simulink model "Robot_Control"  (R2016b)
settings: Solver=ode1  StartTime=0.0  StopTime=Inf  FixedStep=0.001  RelTol=1e-3
PostLoadFcn:
  | , if any(exist('dsrtsu_mdlpostloadfcn', 'file') == [2, 3, 6]), try dsrtsu_mdlpostloadfcn('Execute', bdroot); catch fprintf('Error in PostLoadFcn (dsrtsu_mdlpostloadfcn) for model "%s":\n %s\n', bdroot, lasterr); end, end,
libraries: rtiethernetlib x4
settings Model: DSRTSU_INTERNAL_RTI_VER=490  DSRTSU_INTERNAL_RTI_TYPE=rti1202  Creator=labuser  LastModifiedBy=labuser
settings OptimizationCC: BlockReduction=off  ConditionallyExecuteInputs=off  OptimizeBlockIOStorage=off  BufferReuse=off  GlobalBufferReuse=off  ExpressionFolding=off  LocalBlockOutputs=off
settings HardwareCC: ProdBitPerPointer=32  ProdBitPerSizeT=32  ProdBitPerPtrDiffT=32  ProdLargestAtomicInteger=Integer  ProdEndianess=BigEndian  ProdWordSize=32  ProdHWDeviceType=Custom Processor->Custom  TargetIntDivRoundTo=Zero  TargetEndianess=BigEndian  TargetHWDeviceType=Custom Processor->Custom
settings RTWCC: SystemTargetFile=rti1202.tlc  MakeCommand=make_rti  TemplateMakefile=rti1202.tmf  Description=dSPACE DS1202 Hardware Platform
settings STFCustomTargetCC: ParMdlRefBuildCompliant=on  GRTInterface=off  SystemTargetFile=rti1202.tlc
settings GRTTargetCC: TargetLangStandard=C89/C90 (ANSI)  CompOptLevelCompliant=off  ConcurrentExecutionCompliant=off  CombineOutputUpdateFcns=off  MatFileLogging=off  CPPClassGenCompliant=off  UseToolchainInfoCompliant=off
settings ConfigComp: CovMetricSettings=dswe

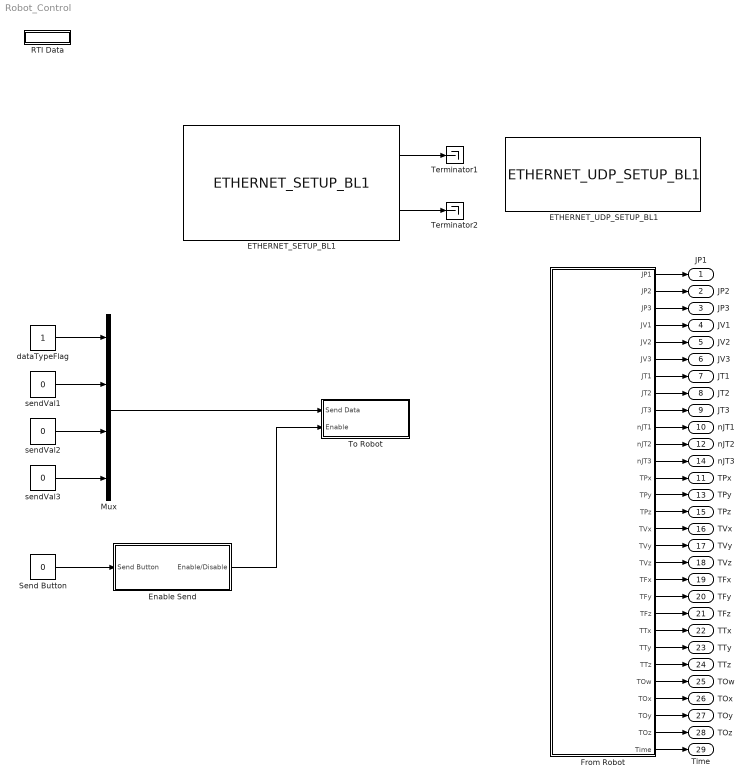
== system Robot_Control ==
  ETHERNET_SETUP_BL1 : rtiethernetlib/ETHERNET_SETUP_BL1  DSProperties=struct('RTI',struct('Version',uint32(2),'BlockType',struct('isSLSource',uint8(0),'isSLSink',uint8(0),'isHWSource',uint8(0),'isHWSink',uint8(0),'isSetup',uint8(1),'isInline',uint8(1),'isNonInline',uint8(0),'isInterrupt',uint8(0),'isChannelwise',uint8(0)),'IOBoardType','DSETHERNET','UnitType','ETHERNET','Identifier','SETUP','DialogType','ML','BlockSet','RTIETHERNET','SlaveProcessor','NONE'))  RTIBlockInterface=struct('OutputPortsWidth',int32([2 1 1 4]),'OutputPortsActive',[0 0 1 1],'OutputPortsName',{{['Link Status'],['Watchdog Status'],['DHCP Status'],['Local IP']}},'OutputPortsDataType',{{'SS_UINT32','SS_UINT32','SS_UINT32','SS_UINT8'}},'InitLevel',3,'IconTransparency','on','BlockDisplay',{{['Ethernet Setup\n\nLocal IP: By DHCP Server'],'left'}},'DialogFcn','rtiethernetsetupgui','BlockName',struct('Token',{{'ETHERNET_SETUP_BL1'}}))  RTIBlockParameters=struct('DHCPserverMode',{{1,'OFF',[0 1]}},'LocalIpNum1',{{'137','OFF',[0 255]}},'LocalIpNum2',{{'148','OFF',[0 255]}},'LocalIpNum3',{{'205','OFF',[0 255]}},'LocalIpNum4',{{'167','OFF',[0 255]}},'SubnetMaskNum1',{{'255','OFF',[0 255]}},'SubnetMaskNum2',{{'255','OFF',[0 255]}},'SubnetMaskNum3',{{'254','OFF',[0 255]}},'SubnetMaskNum4',{{'0','OFF',[0 255]}},'GatewayNum1',{{'0','OFF',[0 255]}},'GatewayNum2',{{'0','OFF',[0 255]}},'GatewayNum3',{{'0','OFF',[0 255]}},'GatewayNum4',{{'0','OFF',[0 255]}},'LinkStatusOutPortMode',{{0,'OFF',[0 1]}},'NumOfEthConnectors',{{2,'ON',[1 16]}},'WatchdogStatusOutPortMode',{{0,'OFF',[0 1]}},'LocalIpOutPortMode',{{1,'OFF',[0 1]}},'IpAndSubmaskCheck',{{int32(0),'OFF',[0 1]}},'TLCFileName',{{'rtiethernetsetup','OFF',[]}})  RTISFcnParameters=struct('DHCPserverMode','int32','LocalIpNum1','uint8','LocalIpNum2','uint8','LocalIpNum3','uint8','LocalIpNum4','uint8','SubnetMaskNum1','uint8','SubnetMaskNum2','uint8','SubnetMaskNum3','uint8','SubnetMaskNum4','uint8','GatewayNum1','uint8','GatewayNum2','uint8','GatewayNum3','uint8','GatewayNum4','uint8','LinkStatusOutPortMode','int32','NumOfEthConnectors','int32','WatchdogStatusOutPortMode','int32','LocalIpOutPortMode','int32','TLCFileName','char')  RTIBlockParaDefault=struct('DHCPserverMode',0,'LocalIpNum1',192,'LocalIpNum2',168,'LocalIpNum3',140,'LocalIpNum4',6,'SubnetMaskNum1',255,'SubnetMaskNum2',255,'SubnetMaskNum3',255,'SubnetMaskNum4',0,'GatewayNum1',0,'GatewayNum2',0,'GatewayNum3',0,'GatewayNum4',0,'LinkStatusOutPortMode',1,'NumOfEthConnectors',3,'WatchdogStatusOutPortMode',0,'LocalIpOutPortMode',0,'IpAndSubmaskCheck',1,'TLCFileName','rtiethernetsetup')
  ETHERNET_UDP_SETUP_BL1 : rtiethernetlib/ETHERNET_UDP_SETUP_BL1  DSProperties=struct('RTI',struct('Version',uint32(2),'BlockType',struct('isSLSource',uint8(1),'isSLSink',uint8(1),'isHWSource',uint8(0),'isHWSink',uint8(0),'isSetup',uint8(0),'isInline',uint8(1),'isNonInline',uint8(0),'isInterrupt',uint8(0),'isChannelwise',uint8(0)),'IOBoardType','DSETHERNET','UnitType','UDP','Identifier','SETUPUDP','DialogType','ML','BlockSet','RTIETHERNET','SlaveProcessor','NONE'))  RTIBlockInterface=struct('OutputPortsWidth',int32(2),'OutputPortsActive',0,'OutputPortsName',{{['RX Dropped Frames']}},'OutputPortsDataType',{{'SS_DOUBLE'}},'InputPortsWidth',int32([4 1]),'InputPortsActive',int32([0 0]),'InputPortsName',{{['RX Remote IP Filter'],['RX Remote Port Filter']}},'InputPortsDataType',{{'SS_UINT8','SS_UINT16'}},'RWork',{{{'RX_DROPPED_FRAMES',uint32(2)}}},'InitLevel',3,'IconTransparency','on','BlockDisplay',{{['Ethernet UDP/IP\nSetup\n\nSocket ID: 0'],'center'}},'DialogFcn','rtiethernetsetupudpgui','BlockName',struct('Token',{{'ETHERNET_UDP_SETUP_BL1'}}))  RTIBlockParameters=struct('SocketId',{{0,'OFF',[]}},'EnableSocketBind',{{1,'OFF',[0 1]}},'AcceptAnyRxRemoteIp',{{1,'OFF',[0 1]}},'RxRemoteIpNum1',{{'172','OFF',[0 255]}},'RxRemoteIpNum2',{{'20','OFF',[0 255]}},'RxRemoteIpNum3',{{'41','OFF',[0 255]}},'RxRemoteIpNum4',{{'226','OFF',[0 255]}},'EnableDynamicRxRemoteIpFilter',{{0,'OFF',[0 1]}},'AcceptAnyRxRemotePort',{{1,'OFF',[0 1]}},'RxRemotePort',{{'9930','OFF',[1 65535]}},'EnableDynamicRxRemotePortFilter',{{0,'OFF',[0 1]}},'TxRemoteIpNum1',{{'137','OFF',[0 255]}},'TxRemoteIpNum2',{{'148','OFF',[0 255]}},'TxRemoteIpNum3',{{'204','OFF',[0 255]}},'TxRemoteIpNum4',{{'55','OFF',[0 255]}},'TxRemotePort',{{'9930','OFF',[1 65535]}},'SpecifyLocalPort',{{1,'OFF',[0 1]}},'LocalPort',{{'9931','OFF',[1 65535]}},'InterruptMode',{{0,'OFF',[0 1]}},'RxDroppedFramesOutPortMode',{{0,'OFF',[0 1]}},'RemoteIpNumCheck',{{0,'OFF',[0 1]}},'RemotePortCheck',{{0,'OFF',[0 1]}},'LocalPortCheck',{{1,'OFF',[0 1]}},'DHCPserverModeEnabled',{{0,'OFF',[0 1]}},'TLCFileName',{{'rtiethernetsetupudp','OFF',[]}})  RTISFcnParameters=struct('SocketId','double','EnableSocketBind','int32','AcceptAnyRxRemoteIp','int32','RxRemoteIpNum1','uint8','RxRemoteIpNum2','uint8','RxRemoteIpNum3','uint8','RxRemoteIpNum4','uint8','EnableDynamicRxRemoteIpFilter','int32','AcceptAnyRxRemotePort','int32','RxRemotePort','uint16','EnableDynamicRxRemotePortFilter','int32','TxRemoteIpNum1','uint8','TxRemoteIpNum2','uint8','TxRemoteIpNum3','uint8','TxRemoteIpNum4','uint8','TxRemotePort','uint16','SpecifyLocalPort','int32','LocalPort','uint16','InterruptMode','int32','RxDroppedFramesOutPortMode','int32','DHCPserverModeEnabled','int32','TLCFileName','char')  RTIBlockParaDefault=struct('SocketId',-1,'EnableSocketBind',1,'AcceptAnyRxRemoteIp',1,'RxRemoteIpNum1',0,'RxRemoteIpNum2',0,'RxRemoteIpNum3',0,'RxRemoteIpNum4',0,'EnableDynamicRxRemoteIpFilter',0,'AcceptAnyRxRemotePort',1,'RxRemotePort',49002,'EnableDynamicRxRemotePortFilter',0,'TxRemoteIpNum1',0,'TxRemoteIpNum2',0,'TxRemoteIpNum3',0,'TxRemoteIpNum4',0,'TxRemotePort',49002,'SpecifyLocalPort',0,'LocalPort',49001,'InterruptMode',0,'RxDroppedFramesOutPortMode',0,'RemoteIpNumCheck',0,'RemotePortCheck',0,'LocalPortCheck',0,'DHCPserverModeEnabled',0,'TLCFileName','rtiethernetsetupudp')
  Enable Send : Subsystem
  From Robot : Subsystem
  Mux : Mux
  RTI Data : Subsystem  Tag=struct('RTIDataServer',struct('RTIDataServerVs','2','RTIModelDescription','struct(''main'',''Robot_Control'',''sub'','''',''isMp'',0)'))  LoadFcn="if exist('rtidc'), try,  rtidc('DataHostBlockClbLoad', gcbh); catch, disp(['Warning: ''LoadFcn'' for RTI Data block failed: ' lasterr]); end, end,"  mask(RTI_DATA_HOST){}
      mask help:
      | RTI Data Block.
      | This block is used by RTI to store internal model-dependent data.
      | Please keep this block on the root level of the model. Deleting this block will result in data loss.
      |
      | NEVER DELETE OR COPY THIS BLOCK!
      settings: CopyFcn="if exist('rtidc'), try,  rtidc('DataHostBlockClbCopy', gcbh); catch, disp(['Warning: ''CopyFcn'' for RTI Data block failed: ' lasterr]); end, end,"  DeleteFcn="if exist('rtidc'), try,  rtidc('DataHostBlockClbDelete', gcbh); catch, disp(['Warning: ''DeleteFcn'' for RTI Data block failed: ' lasterr]); end, end,"  ModelCloseFcn="if exist('rtidc'), try,  rtidc('DataHostBlockClbModelClose', gcbh); catch, disp(['Warning: ''ModelCloseFcn'' for RTI Data block failed: ' lasterr]); end, end,"  PreSaveFcn="if exist('rtidc'), try,  rtidc('DataHostBlockClbPreSave', gcbh); catch, disp(['Warning: ''PreSaveFcn'' for RTI Data block failed: ' lasterr]); end, end,"  PostSaveFcn="if exist('rtidc'), try,  rtidc('DataHostBlockClbPostSave', gcbh); catch, disp(['Warning: ''PostSaveFcn'' for RTI Data block failed: ' lasterr]); end, end,"  NameChangeFcn="if exist('rtidc'), try,  rtidc('DataHostBlockClbNameChange', gcbh); catch, disp(['Warning: ''NameChangeFcn'' for RTI Data block failed: ' lasterr]); end, end,"
      mask Help:
      | RTI Data Block.
      | This block is used by RTI to store internal model-dependent data.
      | Please keep this block on the root level of the model. Deleting this block will result in data loss.
      | 
      | NEVER DELETE OR COPY THIS BLOCK!
      mask Display:
      | text(0.5, 0.5, 'RTI Data', 'HorizontalAlignment', 'center');
      | plot([1 0]);
  Send Button : Constant  Value=0
  Terminator1 : Terminator
  Terminator2 : Terminator
  To Robot : Subsystem
  dataTypeFlag : Constant  Description=|
      | This block determines the data type that the robot controller receives. 
      | If the controller expects a data type different than what you send, it will beep and throw an error.
      | Data Types:
      | 1 - Joint Position
      | 2 - Joint Velocity
      | 3 - Joint Torque (gravity compensated)
      | 4 - Joint Torque (not gravity compensated)
      | 5 - Tool Position
      | 6 - Tool Velocity
  sendVal1 : Constant  Value=0
  sendVal2 : Constant  Value=0
  sendVal3 : Constant  Value=0
  JP1 : Outport
  JP2 : Outport  Port=2
  JP3 : Outport  Port=3
  JV1 : Outport  Port=4
  JV2 : Outport  Port=5
  JV3 : Outport  Port=6
  JT1 : Outport  Port=7
  JT2 : Outport  Port=8
  JT3 : Outport  Port=9
  nJT1 : Outport  Port=10
  TPx : Outport  Port=11
  nJT2 : Outport  Port=12
  TPy : Outport  Port=13
  nJT3 : Outport  Port=14
  TPz : Outport  Port=15
  TVx : Outport  Port=16
  TVy : Outport  Port=17
  TVz : Outport  Port=18
  TFx : Outport  Port=19
  TFy : Outport  Port=20
  TFz : Outport  Port=21
  TTx : Outport  Port=22
  TTy : Outport  Port=23
  TTz : Outport  Port=24
  TOw : Outport  Port=25
  TOx : Outport  Port=26
  TOy : Outport  Port=27
  TOz : Outport  Port=28
  Time : Outport  Port=29
  wires:
  ETHERNET_SETUP_BL1/1 -> Terminator1/1
  ETHERNET_SETUP_BL1/2 -> Terminator2/1
  From Robot/13(TPx) -> TPx/1
  From Robot/14(TPy) -> TPy/1
  From Robot/15(TPz) -> TPz/1
  From Robot/1(JP1) -> JP1/1
  From Robot/2(JP2) -> JP2/1
  From Robot/3(JP3) -> JP3/1
  From Robot/29(Time) -> Time/1
  From Robot/28(TOz) -> TOz/1
  From Robot/27(TOy) -> TOy/1
  From Robot/26(TOx) -> TOx/1
  From Robot/25(TOw) -> TOw/1
  From Robot/24(TTz) -> TTz/1
  From Robot/23(TTy) -> TTy/1
  From Robot/22(TTx) -> TTx/1
  From Robot/21(TFz) -> TFz/1
  From Robot/20(TFy) -> TFy/1
  From Robot/19(TFx) -> TFx/1
  From Robot/18(TVz) -> TVz/1
  From Robot/17(TVy) -> TVy/1
  From Robot/16(TVx) -> TVx/1
  From Robot/12(nJT3) -> nJT3/1
  From Robot/11(nJT2) -> nJT2/1
  From Robot/10(nJT1) -> nJT1/1
  From Robot/9(JT3) -> JT3/1
  From Robot/8(JT2) -> JT2/1
  From Robot/7(JT1) -> JT1/1
  From Robot/6(JV3) -> JV3/1
  From Robot/5(JV2) -> JV2/1
  From Robot/4(JV1) -> JV1/1
  Enable Send/1(Enable/Disable) -> To Robot/2(Enable)
  Send Button/1 -> Enable Send/1(Send Button)
  dataTypeFlag/1 -> Mux/1
  sendVal1/1 -> Mux/2
  sendVal2/1 -> Mux/3
  sendVal3/1 -> Mux/4
  Mux/1 -> To Robot/1(Send Data)

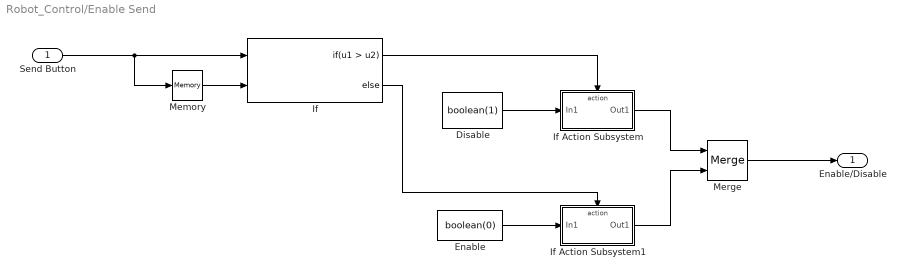
== system Robot_Control/Enable Send ==
  Send Button : Inport
  Disable : Constant  Value=boolean(1)
  Enable : Constant  Value=boolean(0)
  If : If  NumInputs=2  IfExpression=u1 > u2
  If Action Subsystem : Subsystem  TreatAsAtomicUnit=on
  If Action Subsystem1 : Subsystem  TreatAsAtomicUnit=on
  Memory : Memory
  Merge : Merge
  Enable/Disable : Outport
  wires:
  If Action Subsystem1/1(Out1) -> Merge/2
  If/1 -> If Action Subsystem/Action
  If/2 -> If Action Subsystem1/Action
  Send Button/1 -> Memory/1, If/1
  Enable/1 -> If Action Subsystem1/1(In1)
  Memory/1 -> If/2
  Merge/1 -> Enable/Disable/1
  Disable/1 -> If Action Subsystem/1(In1)
  If Action Subsystem/1(Out1) -> Merge/1

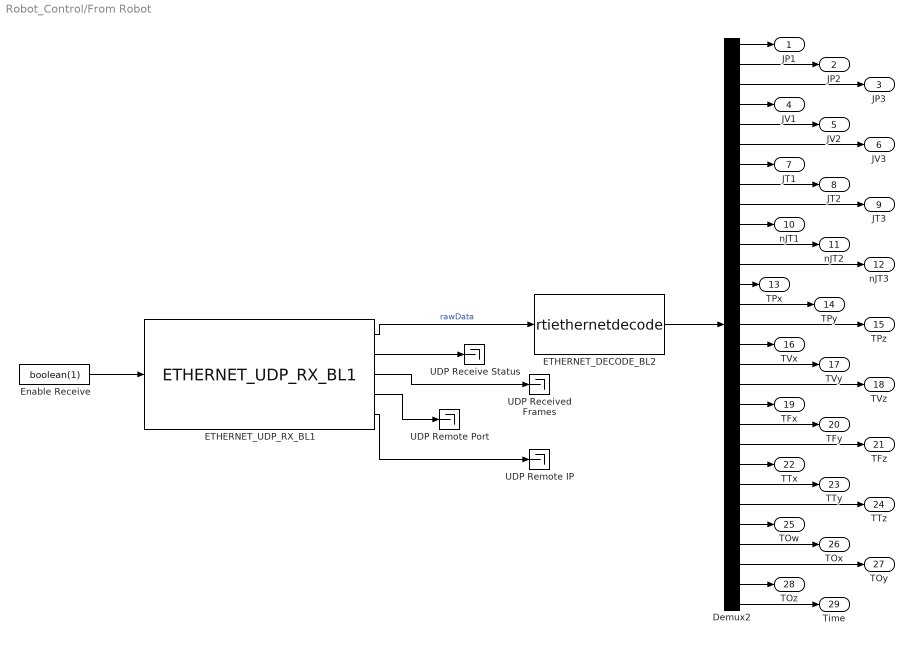
== system Robot_Control/From Robot ==
  Demux2 : Demux  Outputs=29
  ETHERNET_DECODE_BL2 : S-Function  FunctionName=rtiethernetdecode  Parameters=byteordering,offset,auto_offset,datatype,one_datatype,sampletime  SFunctionDeploymentMode=off  EnableBusSupport=off  mask(Ethernet Decode){byteordering=Little endian (Intel), offset=[0], auto_offset=on, datatype=[9 9 9 9 9 9 9 9 9 9 9 9 9 9 9 9 9 9 9 9 9 9 9 9 9 9 9 9 3], one_datatype=off, sampletime=.002}
      mask prompts: byteordering "Byte ordering:"; offset "Offset (bytes):"; auto_offset "Auto offset"; one_datatype "One datatype only"
      mask help:
      | Converts a byte input data stream into the specified datatypes on the output port.
      |
      | Datatype codes:
      | BOOLEAN:  1   //   INT8:      2   //   UINT8:    3
      | INT16  :     4   //   UINT16:  5   //   INT32:     6
      | UINT32 :    7   //   FLOAT:    8   //   DOUBLE:  9
      mask Help: To get further information on this block, refer to the RTI Ethernet blockset documentation.
      mask TypeOptions byteordering: Big endian (Motorola) | Little endian (Intel)
      mask Callback auto_offset: rtiethernetfcnlib('EnableEnDecodeGuiControl', gcbh, 'auto_offset', 2)
      mask Display: text(0.5,0.5, 'Ethernet\nDecode', 'HorizontalAlignment', 'center')
  ETHERNET_UDP_RX_BL1 : rtiethernetlib/ETHERNET_UDP_RX_BL1  DSProperties=struct('RTI',struct('Version',uint32(1),'BlockType',struct('isSLSource',uint8(1),'isSLSink',uint8(1),'isHWSource',uint8(0),'isHWSink',uint8(1),'isSetup',uint8(0),'isInline',uint8(1),'isNonInline',uint8(0),'isInterrupt',uint8(0),'isChannelwise',uint8(0)),'IOBoardType','DSETHERNET','UnitType','UDP','Identifier','RXUDP','DialogType','ML','BlockSet','RTIETHERNET','SlaveProcessor','NONE'))  RTIBlockInterface=struct('OutputPortsWidth',int32([232 1 1 1 4 1]),'OutputPortsActive',[1 1 1 0 1 1],'OutputPortsName',{{'Data','Status',['Received Frames'],['Received Bytes'],['Remote IP'],['Remote Port']}},'OutputPortsDataType',{{'SS_UINT8','SS_UINT32','SS_DOUBLE','SS_UINT32','SS_UINT8','SS_UINT16'}},'InputPortsWidth',int32(1),'InputPortsActive',1,'InputPortsName',{{'Enable'}},'InputPortsDataType',{{'SS_BOOLEAN'}},'RWork',{{{'RECEIVED_FRAMES',uint32(1)}}},'InitLevel',3,'IconTransparency','on','BlockDisplay',{{['Ethernet UDP/IP\nRX\n\nSocket ID: 0'],'center'}},'DialogFcn','rtiethernetrxudpgui','BlockName',struct('Token',{{'ETHERNET_UDP_RX_BL1'}}))  RTIBlockParameters=struct('SocketIdIndex',{{2,'OFF',[1 2]}},'SocketId',{{0,'OFF',[-1 inf]}},'RemoteIp',{{['<NOT AVAILABLE>'],'OFF',[]}},'RemotePort',{{['<NOT AVAILABLE>'],'OFF',[]}},'LocalPort',{{9931,'OFF',[]}},'FrameSize',{{'232','OFF',[1 65507]}},'EnableVariableFrameSize',{{0,'OFF',[0 1]}},'VariableFrameSizeMode',{{1,'OFF',[1 2]}},'InterruptMode',{{0,'OFF',[0 1]}},'RemoteIpOutPortMode',{{1,'OFF',[0 1]}},'RemotePortOutPortMode',{{1,'OFF',[0 1]}},'TLCFileName',{{'rtiethernetrxudp','OFF',[]}})  RTISFcnParameters=struct('SocketIdIndex','int32','SocketId','double','FrameSize','uint16','EnableVariableFrameSize','int32','VariableFrameSizeMode','int32','InterruptMode','int32','RemoteIpOutPortMode','int32','RemotePortOutPortMode','int32','TLCFileName','char')  RTIBlockParaDefault=struct('SocketIdIndex',1,'SocketId',-1,'RemoteIp',['<NOT AVAILABLE>'],'RemotePort',['<NOT AVAILABLE>'],'LocalPort',['<NOT AVAILABLE>'],'FrameSize',1024,'EnableVariableFrameSize',0,'VariableFrameSizeMode',1,'InterruptMode',0,'RemoteIpOutPortMode',0,'RemotePortOutPortMode',0,'TLCFileName','rtiethernetrxudp')
  Enable Receive : Constant  Value=boolean(1)
  UDP Receive Status : Terminator
  UDP Received Frames : Terminator
  UDP Remote IP : Terminator
  UDP Remote Port : Terminator
  JP1 : Outport
  JP2 : Outport  Port=2
  JP3 : Outport  Port=3
  JV1 : Outport  Port=4
  JV2 : Outport  Port=5
  JV3 : Outport  Port=6
  JT1 : Outport  Port=7
  JT2 : Outport  Port=8
  JT3 : Outport  Port=9
  nJT1 : Outport  Port=10
  nJT2 : Outport  Port=11
  nJT3 : Outport  Port=12
  TPx : Outport  Port=13
  TPy : Outport  Port=14
  TPz : Outport  Port=15
  TVx : Outport  Port=16
  TVy : Outport  Port=17
  TVz : Outport  Port=18
  TFx : Outport  Port=19
  TFy : Outport  Port=20
  TFz : Outport  Port=21
  TTx : Outport  Port=22
  TTy : Outport  Port=23
  TTz : Outport  Port=24
  TOw : Outport  Port=25
  TOx : Outport  Port=26
  TOy : Outport  Port=27
  TOz : Outport  Port=28
  Time : Outport  Port=29
  wires:
  ETHERNET_UDP_RX_BL1/2 -> UDP Receive Status/1
  ETHERNET_UDP_RX_BL1/5 -> UDP Remote IP/1
  ETHERNET_UDP_RX_BL1/4 -> UDP Remote Port/1
  ETHERNET_UDP_RX_BL1/1 -> ETHERNET_DECODE_BL2/1  "rawData"
  ETHERNET_UDP_RX_BL1/3 -> UDP Received Frames/1
  Enable Receive/1 -> ETHERNET_UDP_RX_BL1/1
  Demux2/4 -> JV1/1
  Demux2/5 -> JV2/1
  Demux2/6 -> JV3/1
  Demux2/7 -> JT1/1
  Demux2/8 -> JT2/1
  Demux2/9 -> JT3/1
  Demux2/10 -> nJT1/1
  Demux2/11 -> nJT2/1
  Demux2/12 -> nJT3/1
  Demux2/14 -> TPy/1
  Demux2/15 -> TPz/1
  Demux2/16 -> TVx/1
  Demux2/17 -> TVy/1
  Demux2/18 -> TVz/1
  Demux2/19 -> TFx/1
  Demux2/20 -> TFy/1
  Demux2/21 -> TFz/1
  Demux2/22 -> TTx/1
  Demux2/23 -> TTy/1
  Demux2/24 -> TTz/1
  Demux2/1 -> JP1/1
  Demux2/2 -> JP2/1
  Demux2/3 -> JP3/1
  Demux2/25 -> TOw/1
  Demux2/26 -> TOx/1
  Demux2/27 -> TOy/1
  Demux2/28 -> TOz/1
  Demux2/29 -> Time/1
  ETHERNET_DECODE_BL2/1 -> Demux2/1
  Demux2/13 -> TPx/1

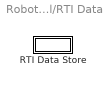
== system Robot_Control/RTI Data ==
  RTI Data Store : Subsystem  Tag="struct('private',struct('version',struct('dsVer',uint32(2),'dsVerCreation',uint32(2),'RTI',struct('ver','7.7','type','RTI1202')),'access',struct('type','Model','isPerm',1,'created',['23-Jan-2020 11:28:27'],'modified',['23-Jan-2020 11:47:49'],'location','')),'public',struct('main',struct('data',[]),'sub',struct('name',{{'Robot_Control'}},'data',{{struct('TH',struct('thTaskInfo',struct('taskType',{'TIMER','HWINT','TMRINT','SWINT','GLINT'},'tasksNumOf',{1,0,0,0,0},'srcIds',{{'TIMERA'},{},{},{},{}},'taskNames',{{['Timer Task 1']},{},{},{},{}})),'th_tc',struct('dataType','TASK','taskGroupId','','taskGroupList',{{}},'taskSchedulingPolicy','FCFS','taskType','TIMER','blkh',-1,'srcId','TIMERA','srcSgnName',['Timer A interrupt'],'srcCpuName','','taskName',['Timer Task 1  [0.001] s'],'taskNameDisplayExt','','smplTime',0.001,'smplTimeOffs',0,'hasFixedPriority',0,'priority',1,'hasFixedOvc',0,'ovcType',1,'ovcMax',1),'tc_th',struct('dataType','TASK','taskGroupId','','taskGroupList',{{}},'taskSchedulingPolicy','FCFS','taskType','TIMER','blkh',-1,'srcId','TIMERA','srcSgnName',['Timer A interrupt'],'srcCpuName','','taskName',['Timer Task 1  [0.001] s'],'taskNameDisplayExt','','smplTime',0.001,'smplTimeOffs',0,'hasFixedPriority',0,'priority',1,'hasFixedOvc',0,'ovcType',1,'ovcMax',1))}})))"  mask(RTI_DATA_STORE){}
      mask help:
      | RTI Data Store Block. This block is used by RTI to store internal model dependent data. Deleting this block will result in data loss.
      |
      | NEVER DELETE, COPY, OR MODIFY THIS BLOCK!
      mask Help:
      | RTI Data Store Block. This block is used by RTI to store internal model dependent data. Deleting this block will result in data loss.
      | 
      | NEVER DELETE, COPY, OR MODIFY THIS BLOCK!
      mask Display: text(0.5, 0.5, ' ', 'HorizontalAlignment', 'center');

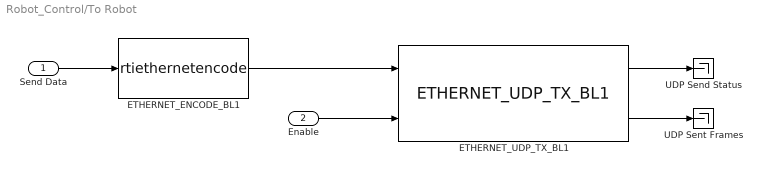
== system Robot_Control/To Robot ==
  Send Data : Inport
  Enable : Inport  Port=2
  ETHERNET_ENCODE_BL1 : S-Function  FunctionName=rtiethernetencode  Parameters=byteordering,offset,auto_offset,datatype,one_datatype,sampletime  SFunctionDeploymentMode=off  EnableBusSupport=off  mask(Ethernet Encode){byteordering=Little endian (Intel), offset=[0], auto_offset=on, datatype=[3 9 9 9], one_datatype=off, sampletime=.002}
      mask prompts: byteordering "Byte ordering:"; offset "Offset (bytes):"; auto_offset "Auto offset"; one_datatype "One datatype only"
      mask help:
      | Converts an input signal consisting of datatypes into a byte data stream on the output port.
      |
      | Datatype codes:
      | BOOLEAN:  1   //   INT8:      2   //   UINT8:    3
      | INT16  :     4   //   UINT16:  5   //   INT32:     6
      | UINT32 :    7   //   FLOAT:    8   //   DOUBLE:  9
      mask Help: To get further information on this block, refer to the RTI Ethernet blockset documentation.
      mask TypeOptions byteordering: Big endian (Motorola) | Little endian (Intel)
      mask Callback auto_offset: rtiethernetfcnlib('EnableEnDecodeGuiControl', gcbh, 'auto_offset', 2)
      mask Display: text(0.5,0.5, 'Ethernet\nEncode', 'HorizontalAlignment', 'center')
  ETHERNET_UDP_TX_BL1 : rtiethernetlib/ETHERNET_UDP_TX_BL1  DSProperties=struct('RTI',struct('Version',uint32(1),'BlockType',struct('isSLSource',uint8(1),'isSLSink',uint8(1),'isHWSource',uint8(0),'isHWSink',uint8(1),'isSetup',uint8(0),'isInline',uint8(1),'isNonInline',uint8(0),'isInterrupt',uint8(0),'isChannelwise',uint8(0)),'IOBoardType','DSETHERNET','UnitType','UDP','Identifier','TXUDP','DialogType','ML','BlockSet','RTIETHERNET','SlaveProcessor','NONE'))  RTIBlockInterface=struct('OutputPortsWidth',int32([1 1]),'OutputPortsActive',[1 1],'OutputPortsName',{{'Status',['Sent Frames']}},'OutputPortsDataType',{{'SS_UINT32','SS_DOUBLE'}},'InputPortsWidth',int32([25 1 1 4 1]),'InputPortsActive',[1 1 0 0 0],'InputPortsName',{{'Data','Enable',['Bytes to Send'],['Remote IP'],['Remote Port']}},'InputPortsDataType',{{'SS_UINT8','SS_BOOLEAN','SS_UINT32','SS_UINT8','SS_UINT16'}},'RWork',{{{'SENT_FRAMES',uint32(1)}}},'InitLevel',3,'IconTransparency','on','BlockDisplay',{{['Ethernet UDP/IP\nTX\n\nSocket ID: 0'],'center'}},'DialogFcn','rtiethernettxudpgui','BlockName',struct('Token',{{'ETHERNET_UDP_TX_BL1'}}))  RTIBlockParameters=struct('SocketIdIndex',{{2,'OFF',[1 2]}},'SocketId',{{0,'OFF',[-1 inf]}},'RemoteIp',{{['<NOT AVAILABLE>'],'OFF',[]}},'RemotePort',{{9930,'OFF',[]}},'LocalPort',{{9931,'OFF',[]}},'EnableDynamicRemoteIp',{{0,'OFF',[0 1]}},'EnableDynamicRemotePort',{{0,'OFF',[0 1]}},'FrameSize',{{'25','OFF',[1 65507]}},'EnableVariableFrameSize',{{0,'OFF',[0 1]}},'SentFramesOutPortMode',{{1,'OFF',[0 1]}},'RemoteIpNum',{{[137 148 204 55],'OFF',[0 255]}},'RemotePortNum',{{9930,'OFF',[0 65535]}},'TLCFileName',{{'rtiethernettxudp','OFF',[]}})  RTISFcnParameters=struct('SocketIdIndex','int32','SocketId','double','EnableDynamicRemoteIp','int32','EnableDynamicRemotePort','int32','FrameSize','uint16','EnableVariableFrameSize','int32','SentFramesOutPortMode','int32','RemoteIpNum','uint8','RemotePortNum','uint16','TLCFileName','char')  RTIBlockParaDefault=struct('SocketIdIndex',1,'SocketId',-1,'RemoteIp',['<NOT AVAILABLE>'],'RemotePort',['<NOT AVAILABLE>'],'LocalPort',['<NOT AVAILABLE>'],'EnableDynamicRemoteIp',0,'EnableDynamicRemotePort',0,'FrameSize',1024,'EnableVariableFrameSize',0,'SentFramesOutPortMode',1,'RemoteIpNum',[0 0 0 0],'RemotePortNum',0,'TLCFileName','rtiethernettxudp')
  UDP Send Status : Terminator
  UDP Sent Frames : Terminator
  wires:
  ETHERNET_UDP_TX_BL1/2 -> UDP Sent Frames/1
  Enable/1 -> ETHERNET_UDP_TX_BL1/2
  Send Data/1 -> ETHERNET_ENCODE_BL1/1
  ETHERNET_ENCODE_BL1/1 -> ETHERNET_UDP_TX_BL1/1
  ETHERNET_UDP_TX_BL1/1 -> UDP Send Status/1

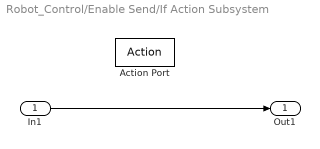
== system Robot_Control/Enable Send/If Action Subsystem ==
  In1 : Inport
  Action Port : ActionPort  ActionType=then
  Out1 : Outport
  wires:
  In1/1 -> Out1/1

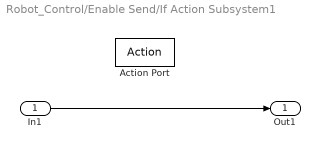
== system Robot_Control/Enable Send/If Action Subsystem1 ==
  In1 : Inport
  Action Port : ActionPort  ActionType=else
  Out1 : Outport
  wires:
  In1/1 -> Out1/1

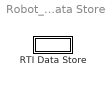
== system Robot_Control/RTI Data/RTI Data Store ==
  RTI Data Store : Subsystem  mask(RTI_DATA_STORE){}
      mask help:
      | RTI Data Store Block. This block is used by RTI to store internal model dependent data. Deleting this block will result in data loss.
      |
      | NEVER DELETE, COPY, OR MODIFY THIS BLOCK!
      mask Help:
      | RTI Data Store Block. This block is used by RTI to store internal model dependent data. Deleting this block will result in data loss.
      | 
      | NEVER DELETE, COPY, OR MODIFY THIS BLOCK!
      mask Display: text(0.5, 0.5, ' ', 'HorizontalAlignment', 'center');

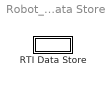
== system Robot_Control/RTI Data/RTI Data Store/RTI Data Store ==
  RTI Data Store : Subsystem  mask(RTI_DATA_STORE){}
      mask help:
      | RTI Data Store Block. This block is used by RTI to store internal model dependent data. Deleting this block will result in data loss.
      |
      | NEVER DELETE, COPY, OR MODIFY THIS BLOCK!
      mask Help:
      | RTI Data Store Block. This block is used by RTI to store internal model dependent data. Deleting this block will result in data loss.
      | 
      | NEVER DELETE, COPY, OR MODIFY THIS BLOCK!
      mask Display: text(0.5, 0.5, ' ', 'HorizontalAlignment', 'center');

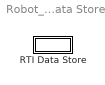
== system Robot_Control/RTI Data/RTI Data Store/RTI Data Store/RTI Data Store ==
  RTI Data Store : Subsystem  mask(RTI_DATA_STORE){}
      mask help:
      | RTI Data Store Block. This block is used by RTI to store internal model dependent data. Deleting this block will result in data loss.
      |
      | NEVER DELETE, COPY, OR MODIFY THIS BLOCK!
      mask Help:
      | RTI Data Store Block. This block is used by RTI to store internal model dependent data. Deleting this block will result in data loss.
      | 
      | NEVER DELETE, COPY, OR MODIFY THIS BLOCK!
      mask Display: text(0.5, 0.5, ' ', 'HorizontalAlignment', 'center');

== system Robot_Control/RTI Data/RTI Data Store/RTI Data Store/RTI Data Store/RTI Data Store ==
